simulink model "BasicRobotV1"  (R2023b)
settings: Solver=VariableStepAuto  StartTime=0.0  StopTime=20.0  RelTol=1e-3
values from neighbouring files (symbols this model uses):
  m = 2.5    [BasicRobot_Parameters.m]
  r = 0.15    [BasicRobot_Parameters.m]
  rr_collide = 0.05    [BasicRobot_Parameters.m]
  rr_stop = 0.21    [BasicRobot_Parameters.m]
  theta0 = deg2rad(theta0_deg)    [BasicRobot_Parameters.m]
  x_obs = 0    [BasicRobot_Parameters.m]
  y_obs = 0    [BasicRobot_Parameters.m]
undefined symbols (not defined in the file or in its folder): magnitude
libraries: simulink x2
settings Model: Creator=BeanieBabyJ  LastModifiedBy=BeanieBabyJ

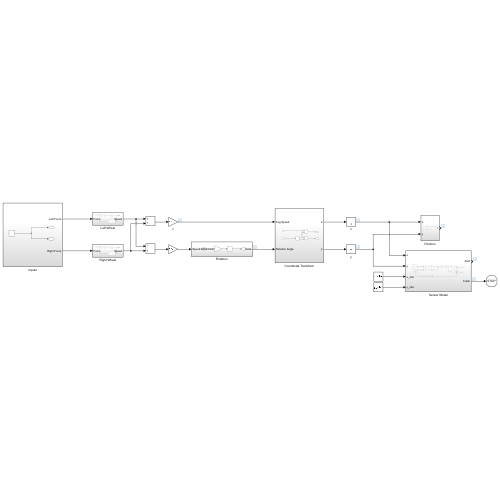
[thumbnail: Simulink's stored preview of the top-level diagram]
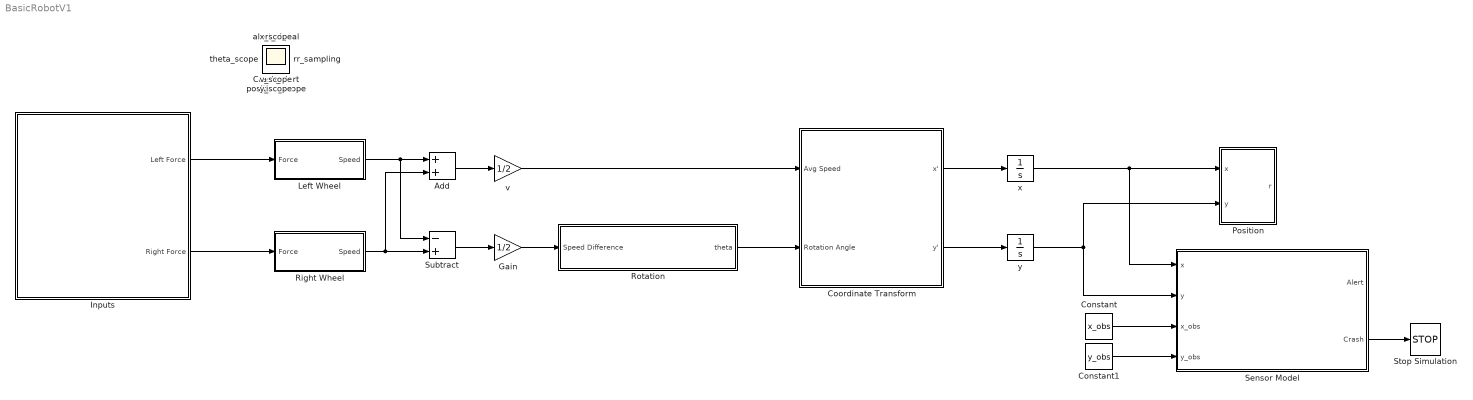
== system BasicRobotV1 ==
  Add : Sum
  Constant : Constant  Value=x_obs
  Constant1 : Constant  Value=y_obs
  Coordinate Transform : Subsystem
  Gain : Gain  Gain=1/2
  Inputs : Subsystem
  Left Wheel : Subsystem
  Position : Subsystem
  Right Wheel : Subsystem
  Rotation : Subsystem
  Sensor Model : Subsystem
  Stop Simulation : Stop
  Subtract : Sum  Inputs=-+
  v : Gain  Gain=1/2
  x : Integrator
  y : Integrator
  Crash_alert : Scope
  alert_signal : Scope
  position_scope : Scope
  rr_sampling : Scope
  theta_scope : Scope
  v_scope : Scope
  x_scope : Scope
  y_scope : Scope
  wires:
  Right Wheel/1(Speed) -> Add/2, Subtract/2
  Left Wheel/1(Speed) -> Add/1, Subtract/1
  Subtract/1 -> Gain/1
  Gain/1 -> Rotation/1(Speed Difference)
  Rotation/1(theta) -> Coordinate Transform/2(Rotation Angle)
  Add/1 -> v/1
  v/1 -> Coordinate Transform/1(Avg Speed)
  Inputs/2(Right Force) -> Right Wheel/1(Force)
  Coordinate Transform/1(x') -> x/1
  Coordinate Transform/2(y') -> y/1
  Inputs/1(Left Force) -> Left Wheel/1(Force)
  x/1 -> Position/1(x), Sensor Model/1(x)
  y/1 -> Position/2(y), Sensor Model/2(y)
  Constant/1 -> Sensor Model/3(x_obs)
  Constant1/1 -> Sensor Model/4(y_obs)
  Sensor Model/2(Crash) -> Stop Simulation/1

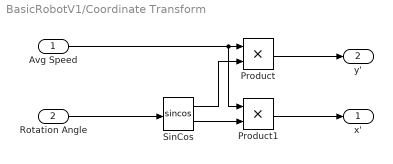
== system BasicRobotV1/Coordinate Transform ==
  Avg Speed : Inport
  Rotation Angle : Inport  Port=2
  Product : Product
  Product1 : Product
  SinCos : Trigonometry  Operator=sincos
  x' : Outport
  y' : Outport  Port=2
  wires:
  Rotation Angle/1 -> SinCos/1
  Avg Speed/1 -> Product1/1, Product/1
  SinCos/1 -> Product/2
  SinCos/2 -> Product1/2
  Product/1 -> y'/1
  Product1/1 -> x'/1

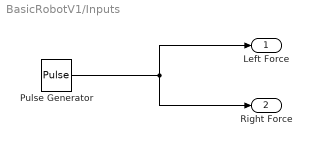
== system BasicRobotV1/Inputs ==
  Pulse Generator : DiscretePulseGenerator  PulseType=Time based  Period=20  PulseWidth=15
  Left Force : Outport
  Right Force : Outport  Port=2
  wires:
  Pulse Generator/1 -> Right Force/1, Left Force/1

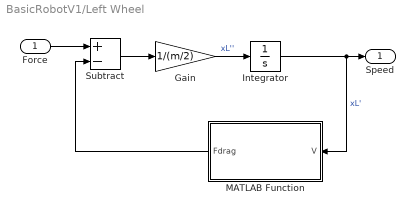
== system BasicRobotV1/Left Wheel ==
  Force : Inport
  Gain : Gain  Gain=1/(m/2)
  Integrator : Integrator
  MATLAB Function : MATLAB Function  TreatAsAtomicUnit=on
  Subtract : Sum  Inputs=+-
  Speed : Outport
  wires:
  Force/1 -> Subtract/1
  MATLAB Function/1(Fdrag) -> Subtract/2
  Subtract/1 -> Gain/1
  Integrator/1 -> MATLAB Function/1(V), Speed/1  "xL'"
  Gain/1 -> Integrator/1  "xL''"

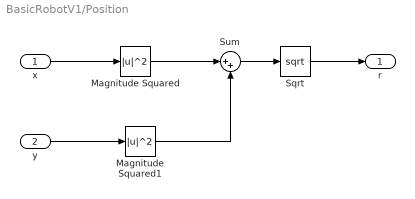
== system BasicRobotV1/Position ==
  x : Inport
  y : Inport  Port=2
  Magnitude Squared : Math  Operator=magnitude^2
  Magnitude Squared1 : Math  Operator=magnitude^2
  Sqrt : Sqrt
  Sum : Sum  Inputs=|++
  r : Outport
  wires:
  Magnitude Squared1/1 -> Sum/2
  Sum/1 -> Sqrt/1
  Magnitude Squared/1 -> Sum/1
  Sqrt/1 -> r/1
  x/1 -> Magnitude Squared/1
  y/1 -> Magnitude Squared1/1

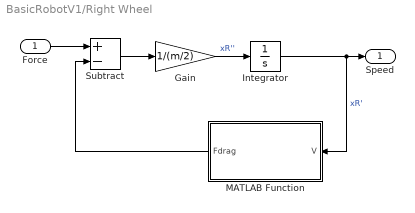
== system BasicRobotV1/Right Wheel ==
  Force : Inport
  Gain : Gain  Gain=1/(m/2)
  Integrator : Integrator
  MATLAB Function : MATLAB Function  TreatAsAtomicUnit=on
  Subtract : Sum  Inputs=+-
  Speed : Outport
  wires:
  Integrator/1 -> MATLAB Function/1(V), Speed/1  "xR'"
  Gain/1 -> Integrator/1  "xR''"
  Force/1 -> Subtract/1
  MATLAB Function/1(Fdrag) -> Subtract/2
  Subtract/1 -> Gain/1

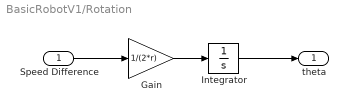
== system BasicRobotV1/Rotation ==
  Speed Difference : Inport
  Gain : Gain  Gain=1/(2*r)
  Integrator : Integrator  InitialCondition=theta0
  theta : Outport
  wires:
  Speed Difference/1 -> Gain/1
  Gain/1 -> Integrator/1
  Integrator/1 -> theta/1

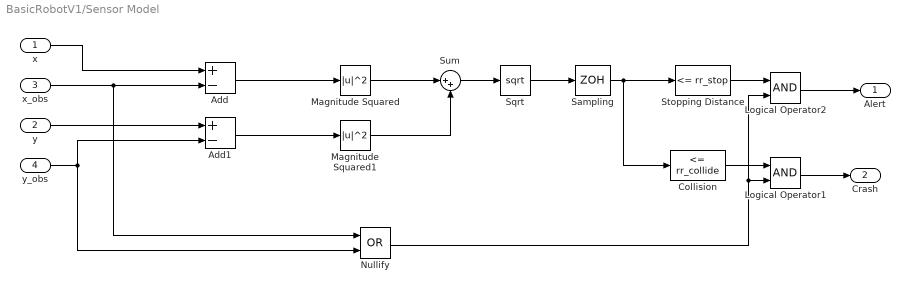
== system BasicRobotV1/Sensor Model ==
  x : Inport
  y : Inport  Port=2
  x_obs : Inport  Port=3
  y_obs : Inport  Port=4
  Add : Sum  Inputs=+-
  Add1 : Sum  Inputs=+-
  Collision : simulink/Logic and Bit Operations/Compare To Constant  relop=<=  const=rr_collide  OutDataTypeStr=boolean
  Logical Operator1 : Logic  AllPortsSameDT=off  OutDataTypeStr=boolean
  Logical Operator2 : Logic  AllPortsSameDT=off  OutDataTypeStr=boolean
  Magnitude Squared : Math  Operator=magnitude^2
  Magnitude Squared1 : Math  Operator=magnitude^2
  Nullify : Logic  Operator=OR  AllPortsSameDT=off  OutDataTypeStr=boolean
  Sampling : ZeroOrderHold  SampleTime=0.25
  Sqrt : Sqrt
  Stopping Distance : simulink/Logic and Bit Operations/Compare To Constant  relop=<=  const=rr_stop  OutDataTypeStr=boolean
  Sum : Sum  Inputs=|++
  Alert : Outport
  Crash : Outport  Port=2
  wires:
  Sampling/1 -> Collision/1, Stopping Distance/1
  x/1 -> Add/1
  Magnitude Squared/1 -> Sum/1
  Sum/1 -> Sqrt/1
  Add/1 -> Magnitude Squared/1
  Add1/1 -> Magnitude Squared1/1
  Sqrt/1 -> Sampling/1
  x_obs/1 -> Nullify/1, Add/2
  y/1 -> Add1/1
  y_obs/1 -> Nullify/2, Add1/2
  Magnitude Squared1/1 -> Sum/2
  Collision/1 -> Logical Operator1/1
  Logical Operator1/1 -> Crash/1
  Nullify/1 -> Logical Operator2/2, Logical Operator1/2
  Stopping Distance/1 -> Logical Operator2/1
  Logical Operator2/1 -> Alert/1

== matlab function BasicRobotV1/Right Wheel/MATLAB Function ==
  data: Fdrag output; V input; k_drag parameter
function Fdrag=get_fdrag(V, k_drag)

Fdrag=k_drag*V*abs(V);

== matlab function BasicRobotV1/Left Wheel/MATLAB Function ==
  data: Fdrag output; V input; k_drag parameter
function Fdrag=get_fdrag(V, k_drag)

Fdrag=k_drag*V*abs(V);
